simulink subsystem "s0330_from_workspace_theta"  (R2019b)
settings: Solver=VariableStepAuto  StartTime=0.0  StopTime=10.0  RelTol=1e-3
undefined symbols (not defined in the file): __PRM__SERIALIZED__DATA__, SubsystemReferenceBlock
settings Model: Creator=paolo  LastModifiedBy=paolo

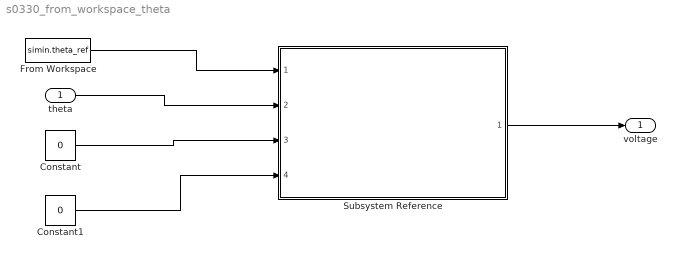
== system s0330_from_workspace_theta ==
  theta : Inport
  Constant : Constant  Value=0
  Constant1 : Constant  Value=0
  From Workspace : FromWorkspace  VariableName=simin.theta_ref  SampleTime=0
  Subsystem Reference : Subsystem  BlockKeywords=__PRM__SERIALIZED__DATA__:SubsystemReferenceBlock  ReferencedSubsystem=s0307_theta_controller_PID  wc=20  cz_ratio=15  pc_ratio=10
  voltage : Outport
  wires:
  Constant1/1 -> Subsystem Reference/4
  Constant/1 -> Subsystem Reference/3
  theta/1 -> Subsystem Reference/2
  From Workspace/1 -> Subsystem Reference/1
  Subsystem Reference/1 -> voltage/1
